simulink model "Test_BadNames"  (R2020a)
settings: configuration reference "testConfig" (kept outside this file)
settings Model: DataDictionary=TestConfig.sldd  Creator=tomha  LastModifiedBy=toma
settings ConfigSetRef: SourceName=testConfig  ParameterOverrideValues=[]

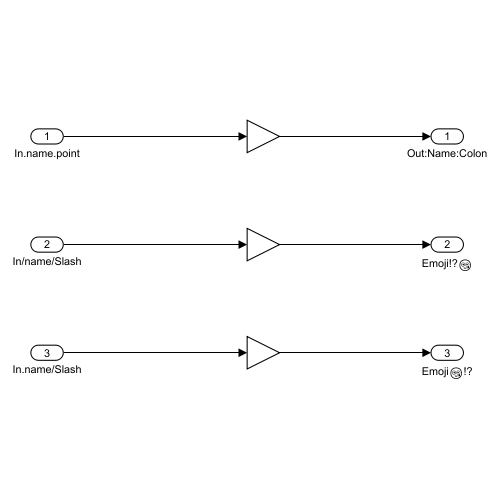
[thumbnail: Simulink's stored preview of the top-level diagram]
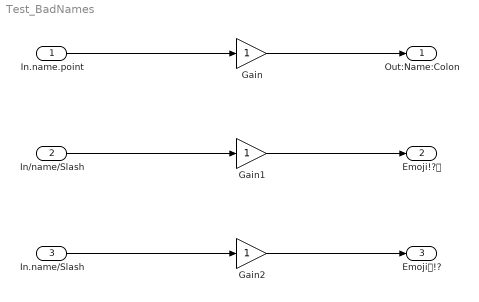
== system Test_BadNames ==
  In.name.point : Inport
  In/name/Slash : Inport  Port=2
  In.name/Slash : Inport  Port=3
  Gain : Gain
  Gain1 : Gain
  Gain2 : Gain
  Out:Name:Colon : Outport
  Emoji!?🥲 : Outport  Port=2
  Emoji🥲!? : Outport  Port=3
  wires:
  Gain/1 -> Out:Name:Colon/1
  In.name.point/1 -> Gain/1
  In/name/Slash/1 -> Gain1/1
  Gain1/1 -> Emoji!?🥲/1
  In.name/Slash/1 -> Gain2/1
  Gain2/1 -> Emoji🥲!?/1
